simulink model "Subsystem"  (R2020b)
settings: Solver=VariableStepAuto  StartTime=0.0  StopTime=10.0  RelTol=1e-3
settings Model: Creator=Akarsh  LastModifiedBy=Akarsh
settings DataIOCC: SaveOutput=off  SaveTime=off

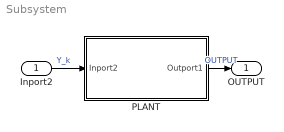
== system Subsystem ==
  Inport2 : Inport  OutDataTypeStr=double  PortDimensions=1  SampleTime=0
  PLANT : Subsystem
  OUTPUT : Outport  OutDataTypeStr=double  PortDimensions=1  SampleTime=0
  wires:
  PLANT/1(Outport1) -> OUTPUT/1  "OUTPUT"
  Inport2/1 -> PLANT/1(Inport2)  "Y_k"

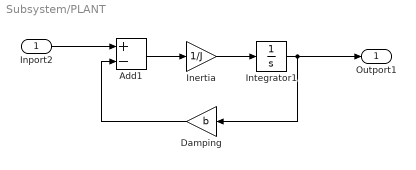
== system Subsystem/PLANT ==
  Inport2 : Inport
  Add1 : Sum  Inputs=+-
  Damping : Gain  Gain=b  mask{b=20, Parameter2=0}
  Inertia : Gain  Gain=1/J  mask{J=100}
  Integrator1 : Integrator
  Outport1 : Outport
  wires:
  Inertia/1 -> Integrator1/1
  Integrator1/1 -> Damping/1, Outport1/1
  Add1/1 -> Inertia/1
  Inport2/1 -> Add1/1
  Damping/1 -> Add1/2
